simulink library "SDTlibV1"  (R2025b)
settings: Solver=VariableStepAuto  StartTime=0.0  StopTime=10.0  RelTol=1e-3
PreLoadFcn:
  | addpath(genpath('SDTfct'));
values from neighbouring files (symbols this model uses):
  pass = ra2DCMi(blk.ra)    [view_SDTlib_model.m]
undefined symbols (not defined in the file or in its folder): CMG, DAP0, DPa0, FSM, Ignew, InvDyn, InvDynAug, Jr, KIN, kinematic_model, LS, Mdyn, mnew, mp, OGnew, PMA, ra_norm, RWS, sig4, uls, ureal, uss, uw, XI
libraries: RCTblocks x470, $bdroot x4
(part 6 of 10)

== system SDTlibV1/Space  subsystems/Four CMGs Pyramid/P2//p' ==
  u : Inport  PortDimensions=18
  Demux : Demux  Outputs=[3 3 3 3 3 3]
  Mux : Mux  Inputs=[3 3 3 3 3 3]
  rotation : Gain  Gain=rot  Multiplication=Matrix(K*u) (u vector)
  rotation1 : Gain  Gain=rot  Multiplication=Matrix(K*u) (u vector)
  rotation2 : Gain  Gain=rot  Multiplication=Matrix(K*u) (u vector)
  translation : Gain  Gain=rot  Multiplication=Matrix(K*u) (u vector)
  translation1 : Gain  Gain=rot  Multiplication=Matrix(K*u) (u vector)
  translation2 : Gain  Gain=rot  Multiplication=Matrix(K*u) (u vector)
  y : Outport  VectorParamsAs1DForOutWhenUnconnected=off
  wires:
  rotation/1 -> Mux/2
  translation/1 -> Mux/1
  Demux/1 -> translation/1
  u/1 -> Demux/1
  Mux/1 -> y/1
  Demux/2 -> rotation/1
  Demux/4 -> rotation1/1
  Demux/3 -> translation1/1
  translation1/1 -> Mux/3
  rotation1/1 -> Mux/4
  Demux/5 -> translation2/1
  translation2/1 -> Mux/5
  rotation2/1 -> Mux/6
  Demux/6 -> rotation2/1

== system SDTlibV1/Space  subsystems/Four CMGs Pyramid/P3//p' ==
  u : Inport  PortDimensions=18
  Demux : Demux  Outputs=[3 3 3 3 3 3]
  Mux : Mux  Inputs=[3 3 3 3 3 3]
  rotation : Gain  Gain=rot  Multiplication=Matrix(K*u) (u vector)
  rotation1 : Gain  Gain=rot  Multiplication=Matrix(K*u) (u vector)
  rotation2 : Gain  Gain=rot  Multiplication=Matrix(K*u) (u vector)
  translation : Gain  Gain=rot  Multiplication=Matrix(K*u) (u vector)
  translation1 : Gain  Gain=rot  Multiplication=Matrix(K*u) (u vector)
  translation2 : Gain  Gain=rot  Multiplication=Matrix(K*u) (u vector)
  y : Outport  VectorParamsAs1DForOutWhenUnconnected=off
  wires:
  Demux/6 -> rotation2/1
  rotation2/1 -> Mux/6
  translation2/1 -> Mux/5
  Demux/5 -> translation2/1
  rotation1/1 -> Mux/4
  translation1/1 -> Mux/3
  Demux/3 -> translation1/1
  Demux/4 -> rotation1/1
  Demux/2 -> rotation/1
  Mux/1 -> y/1
  u/1 -> Demux/1
  Demux/1 -> translation/1
  translation/1 -> Mux/1
  rotation/1 -> Mux/2

== system SDTlibV1/Space  subsystems/Four CMGs Pyramid/P4//p' ==
  u : Inport  PortDimensions=18
  Demux : Demux  Outputs=[3 3 3 3 3 3]
  Mux : Mux  Inputs=[3 3 3 3 3 3]
  rotation : Gain  Gain=rot  Multiplication=Matrix(K*u) (u vector)
  rotation1 : Gain  Gain=rot  Multiplication=Matrix(K*u) (u vector)
  rotation2 : Gain  Gain=rot  Multiplication=Matrix(K*u) (u vector)
  translation : Gain  Gain=rot  Multiplication=Matrix(K*u) (u vector)
  translation1 : Gain  Gain=rot  Multiplication=Matrix(K*u) (u vector)
  translation2 : Gain  Gain=rot  Multiplication=Matrix(K*u) (u vector)
  y : Outport  VectorParamsAs1DForOutWhenUnconnected=off
  wires:
  rotation/1 -> Mux/2
  translation/1 -> Mux/1
  Demux/1 -> translation/1
  u/1 -> Demux/1
  Mux/1 -> y/1
  Demux/2 -> rotation/1
  Demux/4 -> rotation1/1
  Demux/3 -> translation1/1
  translation1/1 -> Mux/3
  rotation1/1 -> Mux/4
  Demux/5 -> translation2/1
  translation2/1 -> Mux/5
  rotation2/1 -> Mux/6
  Demux/6 -> rotation2/1

== system SDTlibV1/Space  subsystems/Four CMGs Pyramid/massless connection body ==
  in1 : Inport  PortDimensions=6
  in2 : Inport  Port=2  PortDimensions=6
  in3 : Inport  Port=3  PortDimensions=6
  in4 : Inport  Port=4  PortDimensions=6
  in5 : Inport  Port=5  PortDimensions=18
  Demux : Demux  Outputs=[ 18 18 18 18 6]
  Gain : RCTblocks/Uncertain State Space  Tag=USS  USystem=uss(KIN)  UValue=[]  X0=[]  uX0=[]
  Mux : Mux  Inputs=[ 6 6 6 6 18]
  out1 : Outport
  out2 : Outport  Port=2
  out3 : Outport  Port=3
  out4 : Outport  Port=4
  out5 : Outport  Port=5
  wires:
  Mux/1 -> Gain/1
  Gain/1 -> Demux/1
  in1/1 -> Mux/1
  Demux/1 -> out1/1
  in2/1 -> Mux/2
  Demux/2 -> out2/1
  in3/1 -> Mux/3
  Demux/3 -> out3/1
  in4/1 -> Mux/4
  Demux/4 -> out4/1
  in5/1 -> Mux/5
  Demux/5 -> out5/1

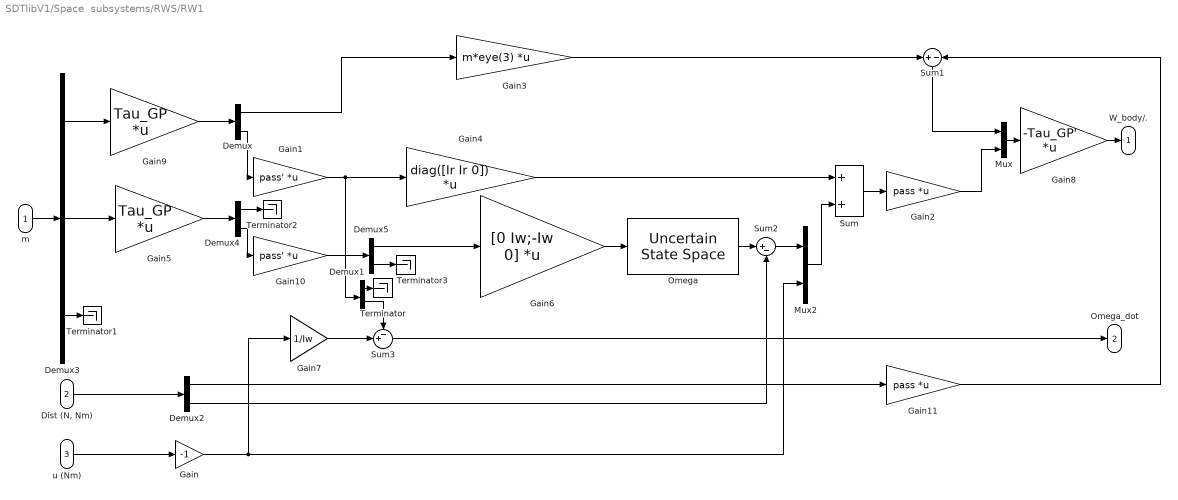
== system SDTlibV1/Space  subsystems/RWS/RW1 ==
  m : Inport  PortDimensions=18
  "Dist (N, Nm)    " : Inport  Port=2
  u (Nm) : Inport  Port=3  PortDimensions=1
  Demux : Demux  Outputs=[3 3]
  Demux1 : Demux  Outputs=[2 1]
  Demux2 : Demux  Outputs=[3 2]
  Demux3 : Demux  Outputs=[6 6 6]
  Demux4 : Demux  Outputs=[3 3]
  Demux5 : Demux  Outputs=[2 1]
  Gain : Gain  Gain=-1
  Gain1 : Gain  Gain=pass'  Multiplication=Matrix(K*u) (u vector)
  Gain10 : Gain  Gain=pass'  Multiplication=Matrix(K*u) (u vector)
  Gain11 : Gain  Gain=pass  Multiplication=Matrix(K*u) (u vector)
  Gain2 : Gain  Gain=pass  Multiplication=Matrix(K*u) (u vector)
  Gain3 : Gain  Gain=m*eye(3)  Multiplication=Matrix(K*u) (u vector)
  Gain4 : Gain  Gain=diag([Ir Ir 0])  Multiplication=Matrix(K*u) (u vector)
  Gain5 : Gain  Gain=Tau_GP  Multiplication=Matrix(K*u) (u vector)
  Gain6 : Gain  Gain=[0 Iw;-Iw 0]  Multiplication=Matrix(K*u) (u vector)
  Gain7 : Gain  Gain=1/Iw
  Gain8 : Gain  Gain=-Tau_GP'  Multiplication=Matrix(K*u) (u vector)
  Gain9 : Gain  Gain=Tau_GP  Multiplication=Matrix(K*u) (u vector)
  Mux : Mux  Inputs=[3 3]
  Mux2 : Mux  Inputs=[2 1]
  Omega : RCTblocks/Uncertain State Space  Tag=USS  USystem=uss(Omega*eye(2))  UValue=[]  X0=[]  uX0=[]
  Sum : Sum
  Sum1 : Sum  Inputs=+-
  Sum2 : Sum  Inputs=|+-
  Sum3 : Sum  Inputs=-+|
  Terminator{,1..3} (4 alike) : Terminator
  W_body/. : Outport  VectorParamsAs1DForOutWhenUnconnected=off
  Omega_dot : Outport  Port=2  PortDimensions=1  VectorParamsAs1DForOutWhenUnconnected=off
  wires:
  Sum3/1 -> Omega_dot/1
  Gain7/1 -> Sum3/2
  Mux2/1 -> Sum/2
  Sum2/1 -> Mux2/1
  Omega/1 -> Sum2/1
  Gain/1 -> Gain7/1, Mux2/2
  u (Nm)/1 -> Gain/1
  Sum1/1 -> Mux/1
  Gain11/1 -> Sum1/2
  Gain3/1 -> Sum1/1
  Demux2/2 -> Sum2/2
  "Dist (N, Nm)    "/1 -> Demux2/1
  Demux2/1 -> Gain11/1
  Gain9/1 -> Demux/1
  Mux/1 -> Gain8/1
  Gain8/1 -> W_body/./1
  Gain6/1 -> Omega/1
  Demux5/1 -> Gain6/1
  Gain1/1 -> Gain4/1, Demux1/1
  Sum/1 -> Gain2/1
  Gain4/1 -> Sum/1
  Demux/2 -> Gain1/1
  Demux/1 -> Gain3/1
  Gain2/1 -> Mux/2
  Demux3/1 -> Gain9/1
  m/1 -> Demux3/1
  Demux3/2 -> Gain5/1
  Demux1/2 -> Sum3/1
  Demux1/1 -> Terminator/1
  Demux3/3 -> Terminator1/1
  Demux4/2 -> Gain10/1
  Gain5/1 -> Demux4/1
  Demux4/1 -> Terminator2/1
  Gain10/1 -> Demux5/1
  Demux5/2 -> Terminator3/1

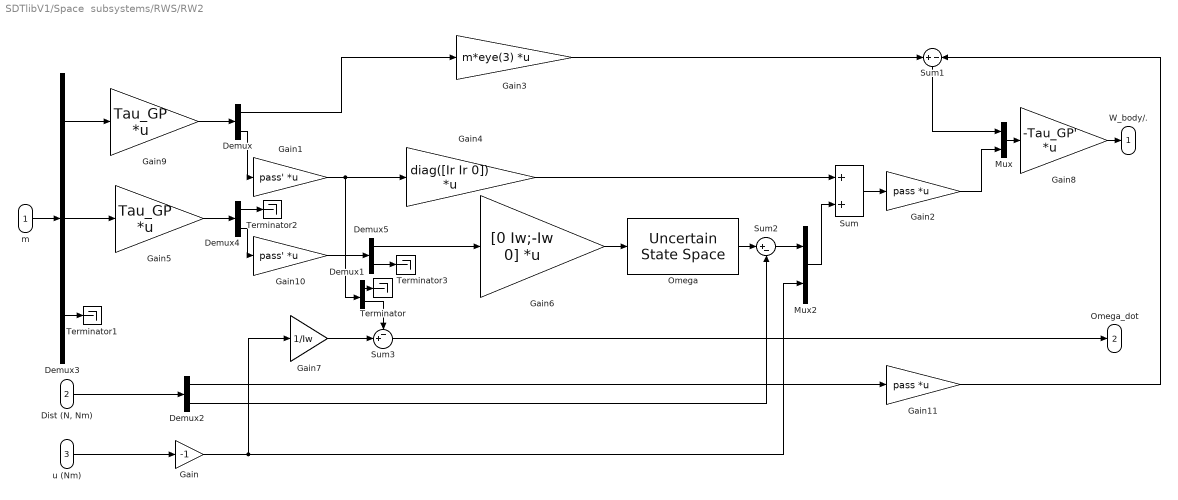
== system SDTlibV1/Space  subsystems/RWS/RW2 ==
  m : Inport  PortDimensions=18
  "Dist (N, Nm)    " : Inport  Port=2
  u (Nm) : Inport  Port=3  PortDimensions=1
  Demux : Demux  Outputs=[3 3]
  Demux1 : Demux  Outputs=[2 1]
  Demux2 : Demux  Outputs=[3 2]
  Demux3 : Demux  Outputs=[6 6 6]
  Demux4 : Demux  Outputs=[3 3]
  Demux5 : Demux  Outputs=[2 1]
  Gain : Gain  Gain=-1
  Gain1 : Gain  Gain=pass'  Multiplication=Matrix(K*u) (u vector)
  Gain10 : Gain  Gain=pass'  Multiplication=Matrix(K*u) (u vector)
  Gain11 : Gain  Gain=pass  Multiplication=Matrix(K*u) (u vector)
  Gain2 : Gain  Gain=pass  Multiplication=Matrix(K*u) (u vector)
  Gain3 : Gain  Gain=m*eye(3)  Multiplication=Matrix(K*u) (u vector)
  Gain4 : Gain  Gain=diag([Ir Ir 0])  Multiplication=Matrix(K*u) (u vector)
  Gain5 : Gain  Gain=Tau_GP  Multiplication=Matrix(K*u) (u vector)
  Gain6 : Gain  Gain=[0 Iw;-Iw 0]  Multiplication=Matrix(K*u) (u vector)
  Gain7 : Gain  Gain=1/Iw
  Gain8 : Gain  Gain=-Tau_GP'  Multiplication=Matrix(K*u) (u vector)
  Gain9 : Gain  Gain=Tau_GP  Multiplication=Matrix(K*u) (u vector)
  Mux : Mux  Inputs=[3 3]
  Mux2 : Mux  Inputs=[2 1]
  Omega : RCTblocks/Uncertain State Space  Tag=USS  USystem=uss(Omega*eye(2))  UValue=[]  X0=[]  uX0=[]
  Sum : Sum
  Sum1 : Sum  Inputs=+-
  Sum2 : Sum  Inputs=|+-
  Sum3 : Sum  Inputs=-+|
  Terminator{,1..3} (4 alike) : Terminator
  W_body/. : Outport  VectorParamsAs1DForOutWhenUnconnected=off
  Omega_dot : Outport  Port=2  PortDimensions=1  VectorParamsAs1DForOutWhenUnconnected=off
  wires:
  Demux5/2 -> Terminator3/1
  Gain10/1 -> Demux5/1
  Demux4/1 -> Terminator2/1
  Gain5/1 -> Demux4/1
  Demux4/2 -> Gain10/1
  Demux3/3 -> Terminator1/1
  Demux1/1 -> Terminator/1
  Demux1/2 -> Sum3/1
  Demux3/2 -> Gain5/1
  m/1 -> Demux3/1
  Demux3/1 -> Gain9/1
  Gain2/1 -> Mux/2
  Demux/1 -> Gain3/1
  Demux/2 -> Gain1/1
  Gain4/1 -> Sum/1
  Sum/1 -> Gain2/1
  Gain1/1 -> Demux1/1, Gain4/1
  Demux5/1 -> Gain6/1
  Gain6/1 -> Omega/1
  Gain8/1 -> W_body/./1
  Mux/1 -> Gain8/1
  Gain9/1 -> Demux/1
  Demux2/1 -> Gain11/1
  "Dist (N, Nm)    "/1 -> Demux2/1
  Demux2/2 -> Sum2/2
  Gain3/1 -> Sum1/1
  Gain11/1 -> Sum1/2
  Sum1/1 -> Mux/1
  u (Nm)/1 -> Gain/1
  Gain/1 -> Mux2/2, Gain7/1
  Omega/1 -> Sum2/1
  Sum2/1 -> Mux2/1
  Mux2/1 -> Sum/2
  Gain7/1 -> Sum3/2
  Sum3/1 -> Omega_dot/1

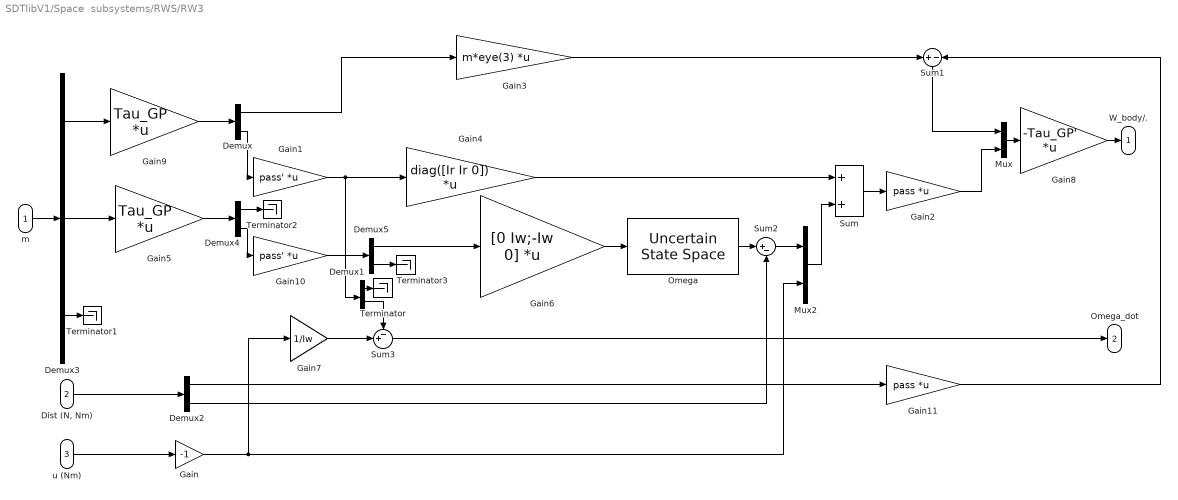
== system SDTlibV1/Space  subsystems/RWS/RW3 ==
  m : Inport  PortDimensions=18
  "Dist (N, Nm)    " : Inport  Port=2
  u (Nm) : Inport  Port=3  PortDimensions=1
  Demux : Demux  Outputs=[3 3]
  Demux1 : Demux  Outputs=[2 1]
  Demux2 : Demux  Outputs=[3 2]
  Demux3 : Demux  Outputs=[6 6 6]
  Demux4 : Demux  Outputs=[3 3]
  Demux5 : Demux  Outputs=[2 1]
  Gain : Gain  Gain=-1
  Gain1 : Gain  Gain=pass'  Multiplication=Matrix(K*u) (u vector)
  Gain10 : Gain  Gain=pass'  Multiplication=Matrix(K*u) (u vector)
  Gain11 : Gain  Gain=pass  Multiplication=Matrix(K*u) (u vector)
  Gain2 : Gain  Gain=pass  Multiplication=Matrix(K*u) (u vector)
  Gain3 : Gain  Gain=m*eye(3)  Multiplication=Matrix(K*u) (u vector)
  Gain4 : Gain  Gain=diag([Ir Ir 0])  Multiplication=Matrix(K*u) (u vector)
  Gain5 : Gain  Gain=Tau_GP  Multiplication=Matrix(K*u) (u vector)
  Gain6 : Gain  Gain=[0 Iw;-Iw 0]  Multiplication=Matrix(K*u) (u vector)
  Gain7 : Gain  Gain=1/Iw
  Gain8 : Gain  Gain=-Tau_GP'  Multiplication=Matrix(K*u) (u vector)
  Gain9 : Gain  Gain=Tau_GP  Multiplication=Matrix(K*u) (u vector)
  Mux : Mux  Inputs=[3 3]
  Mux2 : Mux  Inputs=[2 1]
  Omega : RCTblocks/Uncertain State Space  Tag=USS  USystem=uss(Omega*eye(2))  UValue=[]  X0=[]  uX0=[]
  Sum : Sum
  Sum1 : Sum  Inputs=+-
  Sum2 : Sum  Inputs=|+-
  Sum3 : Sum  Inputs=-+|
  Terminator{,1..3} (4 alike) : Terminator
  W_body/. : Outport  VectorParamsAs1DForOutWhenUnconnected=off
  Omega_dot : Outport  Port=2  PortDimensions=1  VectorParamsAs1DForOutWhenUnconnected=off
  wires:
  Sum3/1 -> Omega_dot/1
  Gain7/1 -> Sum3/2
  Mux2/1 -> Sum/2
  Sum2/1 -> Mux2/1
  Omega/1 -> Sum2/1
  Gain/1 -> Gain7/1, Mux2/2
  u (Nm)/1 -> Gain/1
  Sum1/1 -> Mux/1
  Gain11/1 -> Sum1/2
  Gain3/1 -> Sum1/1
  Demux2/2 -> Sum2/2
  "Dist (N, Nm)    "/1 -> Demux2/1
  Demux2/1 -> Gain11/1
  Gain9/1 -> Demux/1
  Mux/1 -> Gain8/1
  Gain8/1 -> W_body/./1
  Gain6/1 -> Omega/1
  Demux5/1 -> Gain6/1
  Gain1/1 -> Gain4/1, Demux1/1
  Sum/1 -> Gain2/1
  Gain4/1 -> Sum/1
  Demux/2 -> Gain1/1
  Demux/1 -> Gain3/1
  Gain2/1 -> Mux/2
  Demux3/1 -> Gain9/1
  m/1 -> Demux3/1
  Demux3/2 -> Gain5/1
  Demux1/2 -> Sum3/1
  Demux1/1 -> Terminator/1
  Demux3/3 -> Terminator1/1
  Demux4/2 -> Gain10/1
  Gain5/1 -> Demux4/1
  Demux4/1 -> Terminator2/1
  Gain10/1 -> Demux5/1
  Demux5/2 -> Terminator3/1

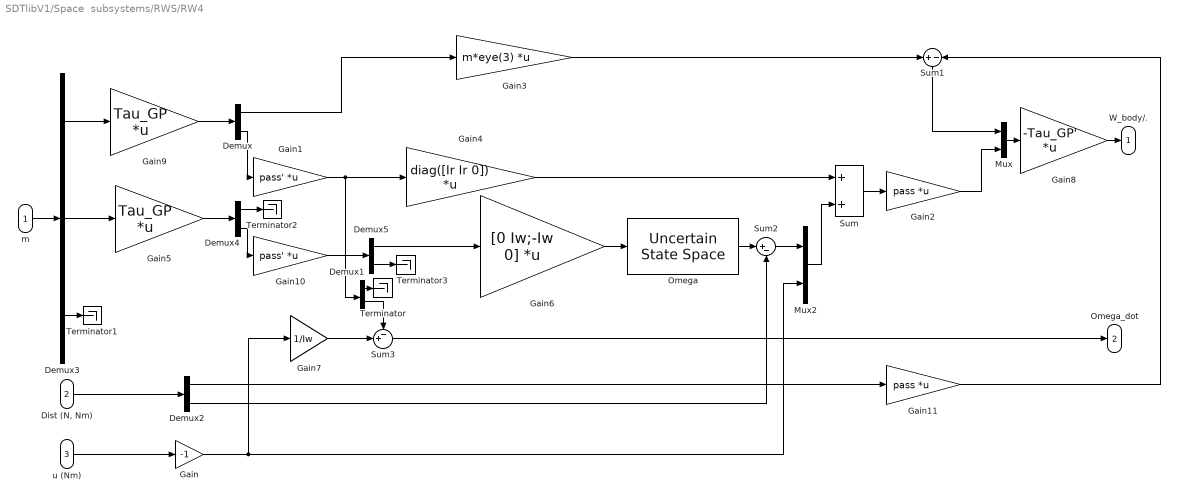
== system SDTlibV1/Space  subsystems/RWS/RW4 ==
  m : Inport  PortDimensions=18
  "Dist (N, Nm)    " : Inport  Port=2
  u (Nm) : Inport  Port=3  PortDimensions=1
  Demux : Demux  Outputs=[3 3]
  Demux1 : Demux  Outputs=[2 1]
  Demux2 : Demux  Outputs=[3 2]
  Demux3 : Demux  Outputs=[6 6 6]
  Demux4 : Demux  Outputs=[3 3]
  Demux5 : Demux  Outputs=[2 1]
  Gain : Gain  Gain=-1
  Gain1 : Gain  Gain=pass'  Multiplication=Matrix(K*u) (u vector)
  Gain10 : Gain  Gain=pass'  Multiplication=Matrix(K*u) (u vector)
  Gain11 : Gain  Gain=pass  Multiplication=Matrix(K*u) (u vector)
  Gain2 : Gain  Gain=pass  Multiplication=Matrix(K*u) (u vector)
  Gain3 : Gain  Gain=m*eye(3)  Multiplication=Matrix(K*u) (u vector)
  Gain4 : Gain  Gain=diag([Ir Ir 0])  Multiplication=Matrix(K*u) (u vector)
  Gain5 : Gain  Gain=Tau_GP  Multiplication=Matrix(K*u) (u vector)
  Gain6 : Gain  Gain=[0 Iw;-Iw 0]  Multiplication=Matrix(K*u) (u vector)
  Gain7 : Gain  Gain=1/Iw
  Gain8 : Gain  Gain=-Tau_GP'  Multiplication=Matrix(K*u) (u vector)
  Gain9 : Gain  Gain=Tau_GP  Multiplication=Matrix(K*u) (u vector)
  Mux : Mux  Inputs=[3 3]
  Mux2 : Mux  Inputs=[2 1]
  Omega : RCTblocks/Uncertain State Space  Tag=USS  USystem=uss(Omega*eye(2))  UValue=[]  X0=[]  uX0=[]
  Sum : Sum
  Sum1 : Sum  Inputs=+-
  Sum2 : Sum  Inputs=|+-
  Sum3 : Sum  Inputs=-+|
  Terminator{,1..3} (4 alike) : Terminator
  W_body/. : Outport  VectorParamsAs1DForOutWhenUnconnected=off
  Omega_dot : Outport  Port=2  PortDimensions=1  VectorParamsAs1DForOutWhenUnconnected=off
  wires:
  Demux5/2 -> Terminator3/1
  Gain10/1 -> Demux5/1
  Demux4/1 -> Terminator2/1
  Gain5/1 -> Demux4/1
  Demux4/2 -> Gain10/1
  Demux3/3 -> Terminator1/1
  Demux1/1 -> Terminator/1
  Demux1/2 -> Sum3/1
  Demux3/2 -> Gain5/1
  m/1 -> Demux3/1
  Demux3/1 -> Gain9/1
  Gain2/1 -> Mux/2
  Demux/1 -> Gain3/1
  Demux/2 -> Gain1/1
  Gain4/1 -> Sum/1
  Sum/1 -> Gain2/1
  Gain1/1 -> Demux1/1, Gain4/1
  Demux5/1 -> Gain6/1
  Gain6/1 -> Omega/1
  Gain8/1 -> W_body/./1
  Mux/1 -> Gain8/1
  Gain9/1 -> Demux/1
  Demux2/1 -> Gain11/1
  "Dist (N, Nm)    "/1 -> Demux2/1
  Demux2/2 -> Sum2/2
  Gain3/1 -> Sum1/1
  Gain11/1 -> Sum1/2
  Sum1/1 -> Mux/1
  u (Nm)/1 -> Gain/1
  Gain/1 -> Mux2/2, Gain7/1
  Omega/1 -> Sum2/1
  Sum2/1 -> Mux2/1
  Mux2/1 -> Sum/2
  Gain7/1 -> Sum3/2
  Sum3/1 -> Omega_dot/1

== system SDTlibV1/Space  subsystems/RWS/massless connection body ==
  in1 : Inport  PortDimensions=18
  in2 : Inport  Port=2  PortDimensions=6
  in3 : Inport  Port=3  PortDimensions=6
  in4 : Inport  Port=4  PortDimensions=6
  in5 : Inport  Port=5  PortDimensions=6
  Demux : Demux  Outputs=[ 6 18 18 18 18]
  Gain : RCTblocks/Uncertain State Space  Tag=USS  USystem=uss(KIN)  UValue=[]  X0=[]  uX0=[]
  Mux : Mux  Inputs=[ 18 6 6 6 6]
  out1 : Outport
  out2 : Outport  Port=2
  out3 : Outport  Port=3
  out4 : Outport  Port=4
  out5 : Outport  Port=5
  wires:
  Mux/1 -> Gain/1
  Gain/1 -> Demux/1
  in1/1 -> Mux/1
  Demux/1 -> out1/1
  in2/1 -> Mux/2
  Demux/2 -> out2/1
  in3/1 -> Mux/3
  Demux/3 -> out3/1
  in4/1 -> Mux/4
  Demux/4 -> out4/1
  in5/1 -> Mux/5
  Demux/5 -> out5/1

== system SDTlibV1/Space  subsystems/Set of 6 PMAss/18x18 DCM ==
  u : Inport  PortDimensions=18
  Demux : Demux  Outputs=[3 3 3 3 3 3]
  Mux : Mux  Inputs=[3 3 3 3 3 3]
  rotation : Gain  Gain=rot  Multiplication=Matrix(K*u) (u vector)
  rotation1 : Gain  Gain=rot  Multiplication=Matrix(K*u) (u vector)
  rotation2 : Gain  Gain=rot  Multiplication=Matrix(K*u) (u vector)
  translation : Gain  Gain=rot  Multiplication=Matrix(K*u) (u vector)
  translation1 : Gain  Gain=rot  Multiplication=Matrix(K*u) (u vector)
  translation2 : Gain  Gain=rot  Multiplication=Matrix(K*u) (u vector)
  y : Outport  VectorParamsAs1DForOutWhenUnconnected=off
  wires:
  rotation/1 -> Mux/2
  translation/1 -> Mux/1
  Demux/1 -> translation/1
  u/1 -> Demux/1
  Mux/1 -> y/1
  Demux/2 -> rotation/1
  Demux/4 -> rotation1/1
  Demux/3 -> translation1/1
  translation1/1 -> Mux/3
  rotation1/1 -> Mux/4
  Demux/5 -> translation2/1
  translation2/1 -> Mux/5
  rotation2/1 -> Mux/6
  Demux/6 -> rotation2/1

== system SDTlibV1/Space  subsystems/Set of 6 PMAss/18x18 DCM1 ==
  u : Inport  PortDimensions=18
  Demux : Demux  Outputs=[3 3 3 3 3 3]
  Mux : Mux  Inputs=[3 3 3 3 3 3]
  rotation : Gain  Gain=rot  Multiplication=Matrix(K*u) (u vector)
  rotation1 : Gain  Gain=rot  Multiplication=Matrix(K*u) (u vector)
  rotation2 : Gain  Gain=rot  Multiplication=Matrix(K*u) (u vector)
  translation : Gain  Gain=rot  Multiplication=Matrix(K*u) (u vector)
  translation1 : Gain  Gain=rot  Multiplication=Matrix(K*u) (u vector)
  translation2 : Gain  Gain=rot  Multiplication=Matrix(K*u) (u vector)
  y : Outport  VectorParamsAs1DForOutWhenUnconnected=off
  wires:
  Demux/6 -> rotation2/1
  rotation2/1 -> Mux/6
  translation2/1 -> Mux/5
  Demux/5 -> translation2/1
  rotation1/1 -> Mux/4
  translation1/1 -> Mux/3
  Demux/3 -> translation1/1
  Demux/4 -> rotation1/1
  Demux/2 -> rotation/1
  Mux/1 -> y/1
  u/1 -> Demux/1
  Demux/1 -> translation/1
  translation/1 -> Mux/1
  rotation/1 -> Mux/2

== system SDTlibV1/Space  subsystems/Set of 6 PMAss/18x18 DCM2 ==
  u : Inport  PortDimensions=18
  Demux : Demux  Outputs=[3 3 3 3 3 3]
  Mux : Mux  Inputs=[3 3 3 3 3 3]
  rotation : Gain  Gain=rot  Multiplication=Matrix(K*u) (u vector)
  rotation1 : Gain  Gain=rot  Multiplication=Matrix(K*u) (u vector)
  rotation2 : Gain  Gain=rot  Multiplication=Matrix(K*u) (u vector)
  translation : Gain  Gain=rot  Multiplication=Matrix(K*u) (u vector)
  translation1 : Gain  Gain=rot  Multiplication=Matrix(K*u) (u vector)
  translation2 : Gain  Gain=rot  Multiplication=Matrix(K*u) (u vector)
  y : Outport  VectorParamsAs1DForOutWhenUnconnected=off
  wires:
  rotation/1 -> Mux/2
  translation/1 -> Mux/1
  Demux/1 -> translation/1
  u/1 -> Demux/1
  Mux/1 -> y/1
  Demux/2 -> rotation/1
  Demux/4 -> rotation1/1
  Demux/3 -> translation1/1
  translation1/1 -> Mux/3
  rotation1/1 -> Mux/4
  Demux/5 -> translation2/1
  translation2/1 -> Mux/5
  rotation2/1 -> Mux/6
  Demux/6 -> rotation2/1

== system SDTlibV1/Space  subsystems/Set of 6 PMAss/6x6 DCM1 ==
  u : Inport  PortDimensions=6
  Demux : Demux  Outputs=[3 3]
  Mux : Mux  Inputs=[3 3]
  rotation : Gain  Gain=rot  Multiplication=Matrix(K*u) (u vector)
  translation : Gain  Gain=rot  Multiplication=Matrix(K*u) (u vector)
  y : Outport  VectorParamsAs1DForOutWhenUnconnected=off
  wires:
  rotation/1 -> Mux/2
  translation/1 -> Mux/1
  Demux/1 -> translation/1
  u/1 -> Demux/1
  Mux/1 -> y/1
  Demux/2 -> rotation/1

== system SDTlibV1/Space  subsystems/Set of 6 PMAss/6x6 DCM2 ==
  u : Inport  PortDimensions=6
  Demux : Demux  Outputs=[3 3]
  Mux : Mux  Inputs=[3 3]
  rotation : Gain  Gain=rot  Multiplication=Matrix(K*u) (u vector)
  translation : Gain  Gain=rot  Multiplication=Matrix(K*u) (u vector)
  y : Outport  VectorParamsAs1DForOutWhenUnconnected=off
  wires:
  rotation/1 -> Mux/2
  translation/1 -> Mux/1
  Demux/1 -> translation/1
  u/1 -> Demux/1
  Mux/1 -> y/1
  Demux/2 -> rotation/1

== system SDTlibV1/Space  subsystems/Set of 6 PMAss/6x6 DCM8 ==
  u : Inport  PortDimensions=6
  Demux : Demux  Outputs=[3 3]
  Mux : Mux  Inputs=[3 3]
  rotation : Gain  Gain=rot  Multiplication=Matrix(K*u) (u vector)
  translation : Gain  Gain=rot  Multiplication=Matrix(K*u) (u vector)
  y : Outport  VectorParamsAs1DForOutWhenUnconnected=off
  wires:
  Demux/2 -> rotation/1
  Mux/1 -> y/1
  u/1 -> Demux/1
  Demux/1 -> translation/1
  translation/1 -> Mux/1
  rotation/1 -> Mux/2

== system SDTlibV1/Space  subsystems/Set of 6 PMAss/PMA1 ==
  m_P : Inport
  u_PMA : Inport  Port=2
  Demux : Demux  Outputs=[6 12]
  Multi port rigid body : Subsystem  mask(Multi-port rigid body (6nx6n)){m=Mc-mp, Ig=IatG, OG=PG, n=2, numinv=1, OP1=[0;0;0], OP2=PG, OP3=[ureal('P3_y',1,'percent',10);0;0], OP4=[0;0;0], OP5=[0;0;0]}
      mask prompts: m "Mass (Kg)"; Ig "Inertia (at G, Kg m^2)"; OG "OG (3x1 vector, m)"; n "Number of ports"; numinv "Port to be inverted"; OP1 "OP1 (3x1 vector, m)"; OP2 "OP2 (3x1 vector, m)"; OP3 "OP3 (3x1 vector, m)"; OP4 "OP4 (3x1 vector, m)"; OP5 "OP5 (3x1 vector,m)"
      mask help:
      | 6nx6n dynamic model of a rigid body at n given points (ports) between wrenches applied at the n points (input) and acceleration twists at these points (output).
      |
      | 0: the reference point
      | G: the center of mass
      | Pi (i=1:n): the n given connection points (n<6).
      |
      | All parameters are expressed in the body frame.
      | Each parameter can be an uncertain parameter declared with "ureal"
      |
      | The 6x6 channel associated to one port can be inverted: then the input of this channel is the acceleration twist imposed at this point and the output is the wrench applied by this body.
      mask init:
      | MultiPortRigidBodyAug
      mask Help: web('Docmultiportrigidbody.html','-browser','-browser')
      mask TypeOptions n: 1 | 2 | 3 | 4 | 5
      mask TypeOptions numinv: 1 | 2 | 3 | 4 | 5
      mask DialogControl ParameterGroupVar Prompt: Main parameters
      mask DialogControl port1 Prompt: Port #1
      mask DialogControl port2 Prompt: #2
      mask DialogControl port3 Prompt: #3
      mask DialogControl port4 Prompt: #4
      mask DialogControl port5 Prompt: #5
      mask Display:
      | disp('Multi-port\n rigid body\n [18(n-1)+6]x[6(n-1)+18])')
      | if n==1,
      |     if numinv==1,
      |         port_label('input', 1,'m_P')
      |         port_label('output',1,'W_body/.,P')
      |     else
      |         port_label('input', 1,'W_./body,P')
      |         port_label('output',1,'m_P')
      |     end
      | else
      |     for ii=1:n
      |         if numinv==ii,
      |             port_label('output',ii,['W_body/.,P',num2str(ii)])
      |             port_label('input', ii,['m_P',num2str(ii)])
      |         else
      |             port_label('input', ii,['W_./body,P',num2str(ii)])
      |             port_label('output',ii,['m_P',num2str(ii)])
      |         end
      |     end
      | end
  Terminator : Terminator
  proof mass : Subsystem  mask(Mass-spring-model model(6x6)){v=v, m=mp, k=k, d=d}
      mask prompts: v "v (3x1 vector)"; m "mass (Kg)"; k "stiffness (N/m)"; d "damper (Ns/m)"
      mask help:
      | Simplified dynamic model of a spring-mass-damper model located at point P (connection point with the hub):
      | 6x6 transfer between acceleretion twist at P and wrench applied by the spring-mass system at P. The model is expressed in the (inherit) body frame.
      |
      | v: the direction vector of the spring-mass system.
      | Each parameter (except v) can be an uncertain parameter declared with "ureal"
      mask init:
      | pass=ra2DCMi(v);
      mask DialogControl ParameterGroupVar Prompt: Main parameters
      mask Display:
      | disp('1D \n mass-spring-damper \n model(6x6)')
      | port_label('input', 1, 'Xddot')
      | port_label('output', 1, 'W_body/.')
      | port_label('input', 2, 'u_PMA')
      | port_label('output', 2, 'x_PMA')
  W_body/.,P : Outport
  x_PMA : Outport  Port=2
  wires:
  Multi port rigid body/1(out1) -> W_body/.,P/1
  u_PMA/1 -> proof mass/2(u_PMA)
  m_P/1 -> Multi port rigid body/1(in1)
  proof mass/1(W_body/.) -> Multi port rigid body/2(in2)
  proof mass/2(x_PMA) -> x_PMA/1
  Multi port rigid body/2(out2) -> Demux/1
  Demux/1 -> proof mass/1(Xddot)
  Demux/2 -> Terminator/1

== system SDTlibV1/Space  subsystems/Set of 6 PMAss/PMA2 ==
  m_P : Inport
  u_PMA : Inport  Port=2
  Demux : Demux  Outputs=[6 12]
  Multi port rigid body : Subsystem  mask(Multi-port rigid body (6nx6n)){m=Mc-mp, Ig=IatG, OG=PG, n=2, numinv=1, OP1=[0;0;0], OP2=PG, OP3=[ureal('P3_y',1,'percent',10);0;0], OP4=[0;0;0], OP5=[0;0;0]}
      mask prompts: m "Mass (Kg)"; Ig "Inertia (at G, Kg m^2)"; OG "OG (3x1 vector, m)"; n "Number of ports"; numinv "Port to be inverted"; OP1 "OP1 (3x1 vector, m)"; OP2 "OP2 (3x1 vector, m)"; OP3 "OP3 (3x1 vector, m)"; OP4 "OP4 (3x1 vector, m)"; OP5 "OP5 (3x1 vector,m)"
      mask help:
      | 6nx6n dynamic model of a rigid body at n given points (ports) between wrenches applied at the n points (input) and acceleration twists at these points (output).
      |
      | 0: the reference point
      | G: the center of mass
      | Pi (i=1:n): the n given connection points (n<6).
      |
      | All parameters are expressed in the body frame.
      | Each parameter can be an uncertain parameter declared with "ureal"
      |
      | The 6x6 channel associated to one port can be inverted: then the input of this channel is the acceleration twist imposed at this point and the output is the wrench applied by this body.
      mask init:
      | MultiPortRigidBodyAug
      mask Help: web('Docmultiportrigidbody.html','-browser','-browser')
      mask TypeOptions n: 1 | 2 | 3 | 4 | 5
      mask TypeOptions numinv: 1 | 2 | 3 | 4 | 5
      mask DialogControl ParameterGroupVar Prompt: Main parameters
      mask DialogControl port1 Prompt: Port #1
      mask DialogControl port2 Prompt: #2
      mask DialogControl port3 Prompt: #3
      mask DialogControl port4 Prompt: #4
      mask DialogControl port5 Prompt: #5
      mask Display:
      | disp('Multi-port\n rigid body\n [18(n-1)+6]x[6(n-1)+18])')
      | if n==1,
      |     if numinv==1,
      |         port_label('input', 1,'m_P')
      |         port_label('output',1,'W_body/.,P')
      |     else
      |         port_label('input', 1,'W_./body,P')
      |         port_label('output',1,'m_P')
      |     end
      | else
      |     for ii=1:n
      |         if numinv==ii,
      |             port_label('output',ii,['W_body/.,P',num2str(ii)])
      |             port_label('input', ii,['m_P',num2str(ii)])
      |         else
      |             port_label('input', ii,['W_./body,P',num2str(ii)])
      |             port_label('output',ii,['m_P',num2str(ii)])
      |         end
      |     end
      | end
  Terminator : Terminator
  proof mass : Subsystem  mask(Mass-spring-model model(6x6)){v=v, m=mp, k=k, d=d}
      mask prompts: v "v (3x1 vector)"; m "mass (Kg)"; k "stiffness (N/m)"; d "damper (Ns/m)"
      mask help:
      | Simplified dynamic model of a spring-mass-damper model located at point P (connection point with the hub):
      | 6x6 transfer between acceleretion twist at P and wrench applied by the spring-mass system at P. The model is expressed in the (inherit) body frame.
      |
      | v: the direction vector of the spring-mass system.
      | Each parameter (except v) can be an uncertain parameter declared with "ureal"
      mask init:
      | pass=ra2DCMi(v);
      mask DialogControl ParameterGroupVar Prompt: Main parameters
      mask Display:
      | disp('1D \n mass-spring-damper \n model(6x6)')
      | port_label('input', 1, 'Xddot')
      | port_label('output', 1, 'W_body/.')
      | port_label('input', 2, 'u_PMA')
      | port_label('output', 2, 'x_PMA')
  W_body/.,P : Outport
  x_PMA : Outport  Port=2
  wires:
  Demux/2 -> Terminator/1
  Demux/1 -> proof mass/1(Xddot)
  Multi port rigid body/2(out2) -> Demux/1
  proof mass/2(x_PMA) -> x_PMA/1
  proof mass/1(W_body/.) -> Multi port rigid body/2(in2)
  m_P/1 -> Multi port rigid body/1(in1)
  u_PMA/1 -> proof mass/2(u_PMA)
  Multi port rigid body/1(out1) -> W_body/.,P/1

== system SDTlibV1/Space  subsystems/Set of 6 PMAss/PMA3 ==
  m_P : Inport
  u_PMA : Inport  Port=2
  Demux : Demux  Outputs=[6 12]
  Multi port rigid body : Subsystem  mask(Multi-port rigid body (6nx6n)){m=Mc-mp, Ig=IatG, OG=PG, n=2, numinv=1, OP1=[0;0;0], OP2=PG, OP3=[ureal('P3_y',1,'percent',10);0;0], OP4=[0;0;0], OP5=[0;0;0]}
      mask prompts: m "Mass (Kg)"; Ig "Inertia (at G, Kg m^2)"; OG "OG (3x1 vector, m)"; n "Number of ports"; numinv "Port to be inverted"; OP1 "OP1 (3x1 vector, m)"; OP2 "OP2 (3x1 vector, m)"; OP3 "OP3 (3x1 vector, m)"; OP4 "OP4 (3x1 vector, m)"; OP5 "OP5 (3x1 vector,m)"
      mask help:
      | 6nx6n dynamic model of a rigid body at n given points (ports) between wrenches applied at the n points (input) and acceleration twists at these points (output).
      |
      | 0: the reference point
      | G: the center of mass
      | Pi (i=1:n): the n given connection points (n<6).
      |
      | All parameters are expressed in the body frame.
      | Each parameter can be an uncertain parameter declared with "ureal"
      |
      | The 6x6 channel associated to one port can be inverted: then the input of this channel is the acceleration twist imposed at this point and the output is the wrench applied by this body.
      mask init:
      | MultiPortRigidBodyAug
      mask Help: web('Docmultiportrigidbody.html','-browser','-browser')
      mask TypeOptions n: 1 | 2 | 3 | 4 | 5
      mask TypeOptions numinv: 1 | 2 | 3 | 4 | 5
      mask DialogControl ParameterGroupVar Prompt: Main parameters
      mask DialogControl port1 Prompt: Port #1
      mask DialogControl port2 Prompt: #2
      mask DialogControl port3 Prompt: #3
      mask DialogControl port4 Prompt: #4
      mask DialogControl port5 Prompt: #5
      mask Display:
      | disp('Multi-port\n rigid body\n [18(n-1)+6]x[6(n-1)+18])')
      | if n==1,
      |     if numinv==1,
      |         port_label('input', 1,'m_P')
      |         port_label('output',1,'W_body/.,P')
      |     else
      |         port_label('input', 1,'W_./body,P')
      |         port_label('output',1,'m_P')
      |     end
      | else
      |     for ii=1:n
      |         if numinv==ii,
      |             port_label('output',ii,['W_body/.,P',num2str(ii)])
      |             port_label('input', ii,['m_P',num2str(ii)])
      |         else
      |             port_label('input', ii,['W_./body,P',num2str(ii)])
      |             port_label('output',ii,['m_P',num2str(ii)])
      |         end
      |     end
      | end
  Terminator : Terminator
  proof mass : Subsystem  mask(Mass-spring-model model(6x6)){v=v, m=mp, k=k, d=d}
      mask prompts: v "v (3x1 vector)"; m "mass (Kg)"; k "stiffness (N/m)"; d "damper (Ns/m)"
      mask help:
      | Simplified dynamic model of a spring-mass-damper model located at point P (connection point with the hub):
      | 6x6 transfer between acceleretion twist at P and wrench applied by the spring-mass system at P. The model is expressed in the (inherit) body frame.
      |
      | v: the direction vector of the spring-mass system.
      | Each parameter (except v) can be an uncertain parameter declared with "ureal"
      mask init:
      | pass=ra2DCMi(v);
      mask DialogControl ParameterGroupVar Prompt: Main parameters
      mask Display:
      | disp('1D \n mass-spring-damper \n model(6x6)')
      | port_label('input', 1, 'Xddot')
      | port_label('output', 1, 'W_body/.')
      | port_label('input', 2, 'u_PMA')
      | port_label('output', 2, 'x_PMA')
  W_body/.,P : Outport
  x_PMA : Outport  Port=2
  wires:
  Multi port rigid body/1(out1) -> W_body/.,P/1
  u_PMA/1 -> proof mass/2(u_PMA)
  m_P/1 -> Multi port rigid body/1(in1)
  proof mass/1(W_body/.) -> Multi port rigid body/2(in2)
  proof mass/2(x_PMA) -> x_PMA/1
  Multi port rigid body/2(out2) -> Demux/1
  Demux/1 -> proof mass/1(Xddot)
  Demux/2 -> Terminator/1

== system SDTlibV1/Space  subsystems/Set of 6 PMAss/PMA4 ==
  m_P : Inport
  u_PMA : Inport  Port=2
  Demux : Demux  Outputs=[6 12]
  Multi port rigid body : Subsystem  mask(Multi-port rigid body (6nx6n)){m=Mc-mp, Ig=IatG, OG=PG, n=2, numinv=1, OP1=[0;0;0], OP2=PG, OP3=[ureal('P3_y',1,'percent',10);0;0], OP4=[0;0;0], OP5=[0;0;0]}
      mask prompts: m "Mass (Kg)"; Ig "Inertia (at G, Kg m^2)"; OG "OG (3x1 vector, m)"; n "Number of ports"; numinv "Port to be inverted"; OP1 "OP1 (3x1 vector, m)"; OP2 "OP2 (3x1 vector, m)"; OP3 "OP3 (3x1 vector, m)"; OP4 "OP4 (3x1 vector, m)"; OP5 "OP5 (3x1 vector,m)"
      mask help:
      | 6nx6n dynamic model of a rigid body at n given points (ports) between wrenches applied at the n points (input) and acceleration twists at these points (output).
      |
      | 0: the reference point
      | G: the center of mass
      | Pi (i=1:n): the n given connection points (n<6).
      |
      | All parameters are expressed in the body frame.
      | Each parameter can be an uncertain parameter declared with "ureal"
      |
      | The 6x6 channel associated to one port can be inverted: then the input of this channel is the acceleration twist imposed at this point and the output is the wrench applied by this body.
      mask init:
      | MultiPortRigidBodyAug
      mask Help: web('Docmultiportrigidbody.html','-browser','-browser')
      mask TypeOptions n: 1 | 2 | 3 | 4 | 5
      mask TypeOptions numinv: 1 | 2 | 3 | 4 | 5
      mask DialogControl ParameterGroupVar Prompt: Main parameters
      mask DialogControl port1 Prompt: Port #1
      mask DialogControl port2 Prompt: #2
      mask DialogControl port3 Prompt: #3
      mask DialogControl port4 Prompt: #4
      mask DialogControl port5 Prompt: #5
      mask Display:
      | disp('Multi-port\n rigid body\n [18(n-1)+6]x[6(n-1)+18])')
      | if n==1,
      |     if numinv==1,
      |         port_label('input', 1,'m_P')
      |         port_label('output',1,'W_body/.,P')
      |     else
      |         port_label('input', 1,'W_./body,P')
      |         port_label('output',1,'m_P')
      |     end
      | else
      |     for ii=1:n
      |         if numinv==ii,
      |             port_label('output',ii,['W_body/.,P',num2str(ii)])
      |             port_label('input', ii,['m_P',num2str(ii)])
      |         else
      |             port_label('input', ii,['W_./body,P',num2str(ii)])
      |             port_label('output',ii,['m_P',num2str(ii)])
      |         end
      |     end
      | end
  Terminator : Terminator
  proof mass : Subsystem  mask(Mass-spring-model model(6x6)){v=v, m=mp, k=k, d=d}
      mask prompts: v "v (3x1 vector)"; m "mass (Kg)"; k "stiffness (N/m)"; d "damper (Ns/m)"
      mask help:
      | Simplified dynamic model of a spring-mass-damper model located at point P (connection point with the hub):
      | 6x6 transfer between acceleretion twist at P and wrench applied by the spring-mass system at P. The model is expressed in the (inherit) body frame.
      |
      | v: the direction vector of the spring-mass system.
      | Each parameter (except v) can be an uncertain parameter declared with "ureal"
      mask init:
      | pass=ra2DCMi(v);
      mask DialogControl ParameterGroupVar Prompt: Main parameters
      mask Display:
      | disp('1D \n mass-spring-damper \n model(6x6)')
      | port_label('input', 1, 'Xddot')
      | port_label('output', 1, 'W_body/.')
      | port_label('input', 2, 'u_PMA')
      | port_label('output', 2, 'x_PMA')
  W_body/.,P : Outport
  x_PMA : Outport  Port=2
  wires:
  Demux/2 -> Terminator/1
  Demux/1 -> proof mass/1(Xddot)
  Multi port rigid body/2(out2) -> Demux/1
  proof mass/2(x_PMA) -> x_PMA/1
  proof mass/1(W_body/.) -> Multi port rigid body/2(in2)
  m_P/1 -> Multi port rigid body/1(in1)
  u_PMA/1 -> proof mass/2(u_PMA)
  Multi port rigid body/1(out1) -> W_body/.,P/1

== system SDTlibV1/Space  subsystems/Set of 6 PMAss/PMA5 ==
  m_P : Inport
  u_PMA : Inport  Port=2
  Demux : Demux  Outputs=[6 12]
  Multi port rigid body : Subsystem  mask(Multi-port rigid body (6nx6n)){m=Mc-mp, Ig=IatG, OG=PG, n=2, numinv=1, OP1=[0;0;0], OP2=PG, OP3=[ureal('P3_y',1,'percent',10);0;0], OP4=[0;0;0], OP5=[0;0;0]}
      mask prompts: m "Mass (Kg)"; Ig "Inertia (at G, Kg m^2)"; OG "OG (3x1 vector, m)"; n "Number of ports"; numinv "Port to be inverted"; OP1 "OP1 (3x1 vector, m)"; OP2 "OP2 (3x1 vector, m)"; OP3 "OP3 (3x1 vector, m)"; OP4 "OP4 (3x1 vector, m)"; OP5 "OP5 (3x1 vector,m)"
      mask help:
      | 6nx6n dynamic model of a rigid body at n given points (ports) between wrenches applied at the n points (input) and acceleration twists at these points (output).
      |
      | 0: the reference point
      | G: the center of mass
      | Pi (i=1:n): the n given connection points (n<6).
      |
      | All parameters are expressed in the body frame.
      | Each parameter can be an uncertain parameter declared with "ureal"
      |
      | The 6x6 channel associated to one port can be inverted: then the input of this channel is the acceleration twist imposed at this point and the output is the wrench applied by this body.
      mask init:
      | MultiPortRigidBodyAug
      mask Help: web('Docmultiportrigidbody.html','-browser','-browser')
      mask TypeOptions n: 1 | 2 | 3 | 4 | 5
      mask TypeOptions numinv: 1 | 2 | 3 | 4 | 5
      mask DialogControl ParameterGroupVar Prompt: Main parameters
      mask DialogControl port1 Prompt: Port #1
      mask DialogControl port2 Prompt: #2
      mask DialogControl port3 Prompt: #3
      mask DialogControl port4 Prompt: #4
      mask DialogControl port5 Prompt: #5
      mask Display:
      | disp('Multi-port\n rigid body\n [18(n-1)+6]x[6(n-1)+18])')
      | if n==1,
      |     if numinv==1,
      |         port_label('input', 1,'m_P')
      |         port_label('output',1,'W_body/.,P')
      |     else
      |         port_label('input', 1,'W_./body,P')
      |         port_label('output',1,'m_P')
      |     end
      | else
      |     for ii=1:n
      |         if numinv==ii,
      |             port_label('output',ii,['W_body/.,P',num2str(ii)])
      |             port_label('input', ii,['m_P',num2str(ii)])
      |         else
      |             port_label('input', ii,['W_./body,P',num2str(ii)])
      |             port_label('output',ii,['m_P',num2str(ii)])
      |         end
      |     end
      | end
  Terminator : Terminator
  proof mass : Subsystem  mask(Mass-spring-model model(6x6)){v=v, m=mp, k=k, d=d}
      mask prompts: v "v (3x1 vector)"; m "mass (Kg)"; k "stiffness (N/m)"; d "damper (Ns/m)"
      mask help:
      | Simplified dynamic model of a spring-mass-damper model located at point P (connection point with the hub):
      | 6x6 transfer between acceleretion twist at P and wrench applied by the spring-mass system at P. The model is expressed in the (inherit) body frame.
      |
      | v: the direction vector of the spring-mass system.
      | Each parameter (except v) can be an uncertain parameter declared with "ureal"
      mask init:
      | pass=ra2DCMi(v);
      mask DialogControl ParameterGroupVar Prompt: Main parameters
      mask Display:
      | disp('1D \n mass-spring-damper \n model(6x6)')
      | port_label('input', 1, 'Xddot')
      | port_label('output', 1, 'W_body/.')
      | port_label('input', 2, 'u_PMA')
      | port_label('output', 2, 'x_PMA')
  W_body/.,P : Outport
  x_PMA : Outport  Port=2
  wires:
  Multi port rigid body/1(out1) -> W_body/.,P/1
  u_PMA/1 -> proof mass/2(u_PMA)
  m_P/1 -> Multi port rigid body/1(in1)
  proof mass/1(W_body/.) -> Multi port rigid body/2(in2)
  proof mass/2(x_PMA) -> x_PMA/1
  Multi port rigid body/2(out2) -> Demux/1
  Demux/1 -> proof mass/1(Xddot)
  Demux/2 -> Terminator/1

== system SDTlibV1/Space  subsystems/Set of 6 PMAss/PMA6 ==
  m_P : Inport
  u_PMA : Inport  Port=2
  Demux : Demux  Outputs=[6 12]
  Multi port rigid body : Subsystem  mask(Multi-port rigid body (6nx6n)){m=Mc-mp, Ig=IatG, OG=PG, n=2, numinv=1, OP1=[0;0;0], OP2=PG, OP3=[ureal('P3_y',1,'percent',10);0;0], OP4=[0;0;0], OP5=[0;0;0]}
      mask prompts: m "Mass (Kg)"; Ig "Inertia (at G, Kg m^2)"; OG "OG (3x1 vector, m)"; n "Number of ports"; numinv "Port to be inverted"; OP1 "OP1 (3x1 vector, m)"; OP2 "OP2 (3x1 vector, m)"; OP3 "OP3 (3x1 vector, m)"; OP4 "OP4 (3x1 vector, m)"; OP5 "OP5 (3x1 vector,m)"
      mask help:
      | 6nx6n dynamic model of a rigid body at n given points (ports) between wrenches applied at the n points (input) and acceleration twists at these points (output).
      |
      | 0: the reference point
      | G: the center of mass
      | Pi (i=1:n): the n given connection points (n<6).
      |
      | All parameters are expressed in the body frame.
      | Each parameter can be an uncertain parameter declared with "ureal"
      |
      | The 6x6 channel associated to one port can be inverted: then the input of this channel is the acceleration twist imposed at this point and the output is the wrench applied by this body.
      mask init:
      | MultiPortRigidBodyAug
      mask Help: web('Docmultiportrigidbody.html','-browser','-browser')
      mask TypeOptions n: 1 | 2 | 3 | 4 | 5
      mask TypeOptions numinv: 1 | 2 | 3 | 4 | 5
      mask DialogControl ParameterGroupVar Prompt: Main parameters
      mask DialogControl port1 Prompt: Port #1
      mask DialogControl port2 Prompt: #2
      mask DialogControl port3 Prompt: #3
      mask DialogControl port4 Prompt: #4
      mask DialogControl port5 Prompt: #5
      mask Display:
      | disp('Multi-port\n rigid body\n [18(n-1)+6]x[6(n-1)+18])')
      | if n==1,
      |     if numinv==1,
      |         port_label('input', 1,'m_P')
      |         port_label('output',1,'W_body/.,P')
      |     else
      |         port_label('input', 1,'W_./body,P')
      |         port_label('output',1,'m_P')
      |     end
      | else
      |     for ii=1:n
      |         if numinv==ii,
      |             port_label('output',ii,['W_body/.,P',num2str(ii)])
      |             port_label('input', ii,['m_P',num2str(ii)])
      |         else
      |             port_label('input', ii,['W_./body,P',num2str(ii)])
      |             port_label('output',ii,['m_P',num2str(ii)])
      |         end
      |     end
      | end
  Terminator : Terminator
  proof mass : Subsystem  mask(Mass-spring-model model(6x6)){v=v, m=mp, k=k, d=d}
      mask prompts: v "v (3x1 vector)"; m "mass (Kg)"; k "stiffness (N/m)"; d "damper (Ns/m)"
      mask help:
      | Simplified dynamic model of a spring-mass-damper model located at point P (connection point with the hub):
      | 6x6 transfer between acceleretion twist at P and wrench applied by the spring-mass system at P. The model is expressed in the (inherit) body frame.
      |
      | v: the direction vector of the spring-mass system.
      | Each parameter (except v) can be an uncertain parameter declared with "ureal"
      mask init:
      | pass=ra2DCMi(v);
      mask DialogControl ParameterGroupVar Prompt: Main parameters
      mask Display:
      | disp('1D \n mass-spring-damper \n model(6x6)')
      | port_label('input', 1, 'Xddot')
      | port_label('output', 1, 'W_body/.')
      | port_label('input', 2, 'u_PMA')
      | port_label('output', 2, 'x_PMA')
  W_body/.,P : Outport
  x_PMA : Outport  Port=2
  wires:
  Demux/2 -> Terminator/1
  Demux/1 -> proof mass/1(Xddot)
  Multi port rigid body/2(out2) -> Demux/1
  proof mass/2(x_PMA) -> x_PMA/1
  proof mass/1(W_body/.) -> Multi port rigid body/2(in2)
  m_P/1 -> Multi port rigid body/1(in1)
  u_PMA/1 -> proof mass/2(u_PMA)
  Multi port rigid body/1(out1) -> W_body/.,P/1

== system SDTlibV1/Space  subsystems/Set of 6 PMAss/massless connection body ==
  in1 : Inport  PortDimensions=18
  in2 : Inport  Port=2  PortDimensions=6
  in3 : Inport  Port=3  PortDimensions=6
  in4 : Inport  Port=4  PortDimensions=6
  in5 : Inport  Port=5  PortDimensions=6
  in6 : Inport  Port=6  PortDimensions=6
  in7 : Inport  Port=7  PortDimensions=6
  Demux : Demux  Outputs=[ 6 18 18 18 18 18 18]
  Gain : RCTblocks/Uncertain State Space  Tag=USS  USystem=uss(KIN)  UValue=[]  X0=[]  uX0=[]
  Mux : Mux  Inputs=[ 18 6 6 6 6 6 6]
  out1 : Outport
  out2 : Outport  Port=2
  out3 : Outport  Port=3
  out4 : Outport  Port=4
  out5 : Outport  Port=5
  out6 : Outport  Port=6
  out7 : Outport  Port=7
  wires:
  Mux/1 -> Gain/1
  Gain/1 -> Demux/1
  in1/1 -> Mux/1
  Demux/1 -> out1/1
  in2/1 -> Mux/2
  Demux/2 -> out2/1
  in3/1 -> Mux/3
  Demux/3 -> out3/1
  in4/1 -> Mux/4
  Demux/4 -> out4/1
  in5/1 -> Mux/5
  Demux/5 -> out5/1
  in6/1 -> Mux/6
  Demux/6 -> out6/1
  in7/1 -> Mux/7
  Demux/7 -> out7/1

== system SDTlibV1/6 dof mechanisms/Revolute joint + configuration/18x18 v-u_rotation/Subsystem ==
  In1 : Inport
  Demux : Demux  Outputs=3
  Gain : Gain  Gain=2
  Gain1 : Gain  Gain=-2
  Gain2 : Gain  Gain=2
  Gain3 : Gain  Gain=2
  Gain4 : Gain  Gain=pass  Multiplication=Matrix(K*u) (u vector)
  Gain5 : Gain  Gain=pass'  Multiplication=Matrix(K*u) (u vector)
  Mux : Mux  Inputs=3
  Sum : Sum  Inputs=++|
  Sum1 : Sum  Inputs=|++
  Sum2 : Sum  Inputs=|+-
  Sum3 : Sum  Inputs=|++
  Sum4 : Sum  Inputs=++|
  Sum5 : Sum  Inputs=++|
  Uncertain State Space{,1..3} (4 alike) : RCTblocks/Uncertain State Space  Tag=USS  USystem=uss(sig4)  UValue=[]  X0=[]  uX0=[]
  Out1 : Outport  VectorParamsAs1DForOutWhenUnconnected=off
  wires:
  Gain5/1 -> Demux/1
  Gain4/1 -> Out1/1
  Uncertain State Space3/1 -> Sum3/2
  Gain2/1 -> Sum3/1
  In1/1 -> Gain5/1
  Gain/1 -> Sum/2
  Uncertain State Space2/1 -> Uncertain State Space3/1, Sum4/2, Sum2/2
  Demux/1 -> Gain3/1, Sum1/2
  Demux/3 -> Mux/3
  Mux/1 -> Gain4/1
  Sum4/1 -> Mux/2
  Sum3/1 -> Uncertain State Space2/1
  Gain1/1 -> Sum2/1
  Uncertain State Space/1 -> Uncertain State Space1/1, Sum5/1, Sum1/1
  Gain3/1 -> Sum5/2
  Sum/1 -> Uncertain State Space/1
  Demux/2 -> Sum4/1, Gain1/1
  Uncertain State Space1/1 -> Sum/1
  Sum2/1 -> Gain/1
  Sum1/1 -> Mux/1
  Sum5/1 -> Gain2/1

== system SDTlibV1/6 dof mechanisms/Revolute joint + configuration/18x18 v-u_rotation/Subsystem1 ==
  In1 : Inport
  Demux : Demux  Outputs=3
  Gain : Gain  Gain=2
  Gain1 : Gain  Gain=-2
  Gain2 : Gain  Gain=2
  Gain3 : Gain  Gain=2
  Gain4 : Gain  Gain=pass  Multiplication=Matrix(K*u) (u vector)
  Gain5 : Gain  Gain=pass'  Multiplication=Matrix(K*u) (u vector)
  Mux : Mux  Inputs=3
  Sum : Sum  Inputs=++|
  Sum1 : Sum  Inputs=|++
  Sum2 : Sum  Inputs=|+-
  Sum3 : Sum  Inputs=|++
  Sum4 : Sum  Inputs=++|
  Sum5 : Sum  Inputs=++|
  Uncertain State Space{,1..3} (4 alike) : RCTblocks/Uncertain State Space  Tag=USS  USystem=uss(sig4)  UValue=[]  X0=[]  uX0=[]
  Out1 : Outport  VectorParamsAs1DForOutWhenUnconnected=off
  wires:
  Gain5/1 -> Demux/1
  Sum5/1 -> Gain2/1
  Sum1/1 -> Mux/1
  Sum2/1 -> Gain/1
  Uncertain State Space1/1 -> Sum/1
  Demux/2 -> Gain1/1, Sum4/1
  Sum/1 -> Uncertain State Space/1
  Gain3/1 -> Sum5/2
  Uncertain State Space/1 -> Sum1/1, Sum5/1, Uncertain State Space1/1
  Gain1/1 -> Sum2/1
  Sum3/1 -> Uncertain State Space2/1
  Sum4/1 -> Mux/2
  Mux/1 -> Gain4/1
  Demux/3 -> Mux/3
  Demux/1 -> Sum1/2, Gain3/1
  Uncertain State Space2/1 -> Sum2/2, Sum4/2, Uncertain State Space3/1
  Gain/1 -> Sum/2
  In1/1 -> Gain5/1
  Gain2/1 -> Sum3/1
  Uncertain State Space3/1 -> Sum3/2
  Gain4/1 -> Out1/1

== system SDTlibV1/6 dof mechanisms/Revolute joint + configuration/18x18 v-u_rotation/Subsystem2 ==
  In1 : Inport
  Demux : Demux  Outputs=3
  Gain : Gain  Gain=2
  Gain1 : Gain  Gain=-2
  Gain2 : Gain  Gain=2
  Gain3 : Gain  Gain=2
  Gain4 : Gain  Gain=pass  Multiplication=Matrix(K*u) (u vector)
  Gain5 : Gain  Gain=pass'  Multiplication=Matrix(K*u) (u vector)
  Mux : Mux  Inputs=3
  Sum : Sum  Inputs=++|
  Sum1 : Sum  Inputs=|++
  Sum2 : Sum  Inputs=|+-
  Sum3 : Sum  Inputs=|++
  Sum4 : Sum  Inputs=++|
  Sum5 : Sum  Inputs=++|
  Uncertain State Space{,1..3} (4 alike) : RCTblocks/Uncertain State Space  Tag=USS  USystem=uss(sig4)  UValue=[]  X0=[]  uX0=[]
  Out1 : Outport  VectorParamsAs1DForOutWhenUnconnected=off
  wires:
  Sum5/1 -> Gain2/1
  Sum1/1 -> Mux/1
  Sum2/1 -> Gain/1
  Uncertain State Space1/1 -> Sum/1
  Demux/2 -> Gain1/1, Sum4/1
  Sum/1 -> Uncertain State Space/1
  Gain3/1 -> Sum5/2
  Uncertain State Space/1 -> Sum1/1, Sum5/1, Uncertain State Space1/1
  Gain1/1 -> Sum2/1
  Sum3/1 -> Uncertain State Space2/1
  Sum4/1 -> Mux/2
  Mux/1 -> Gain4/1
  Demux/3 -> Mux/3
  Demux/1 -> Sum1/2, Gain3/1
  Uncertain State Space2/1 -> Sum2/2, Sum4/2, Uncertain State Space3/1
  Gain/1 -> Sum/2
  In1/1 -> Gain5/1
  Gain2/1 -> Sum3/1
  Uncertain State Space3/1 -> Sum3/2
  Gain4/1 -> Out1/1
  Gain5/1 -> Demux/1

== system SDTlibV1/6 dof mechanisms/Revolute joint + configuration/18x18 v-u_rotation/Subsystem3 ==
  In1 : Inport
  Demux : Demux  Outputs=3
  Gain : Gain  Gain=2
  Gain1 : Gain  Gain=-2
  Gain2 : Gain  Gain=2
  Gain3 : Gain  Gain=2
  Gain4 : Gain  Gain=pass  Multiplication=Matrix(K*u) (u vector)
  Gain5 : Gain  Gain=pass'  Multiplication=Matrix(K*u) (u vector)
  Mux : Mux  Inputs=3
  Sum : Sum  Inputs=++|
  Sum1 : Sum  Inputs=|++
  Sum2 : Sum  Inputs=|+-
  Sum3 : Sum  Inputs=|++
  Sum4 : Sum  Inputs=++|
  Sum5 : Sum  Inputs=++|
  Uncertain State Space{,1..3} (4 alike) : RCTblocks/Uncertain State Space  Tag=USS  USystem=uss(sig4)  UValue=[]  X0=[]  uX0=[]
  Out1 : Outport  VectorParamsAs1DForOutWhenUnconnected=off
  wires:
  Gain4/1 -> Out1/1
  Uncertain State Space3/1 -> Sum3/2
  Gain2/1 -> Sum3/1
  In1/1 -> Gain5/1
  Gain/1 -> Sum/2
  Uncertain State Space2/1 -> Uncertain State Space3/1, Sum4/2, Sum2/2
  Demux/1 -> Gain3/1, Sum1/2
  Demux/3 -> Mux/3
  Mux/1 -> Gain4/1
  Sum4/1 -> Mux/2
  Sum3/1 -> Uncertain State Space2/1
  Gain1/1 -> Sum2/1
  Uncertain State Space/1 -> Uncertain State Space1/1, Sum5/1, Sum1/1
  Gain3/1 -> Sum5/2
  Sum/1 -> Uncertain State Space/1
  Demux/2 -> Sum4/1, Gain1/1
  Uncertain State Space1/1 -> Sum/1
  Sum2/1 -> Gain/1
  Sum1/1 -> Mux/1
  Sum5/1 -> Gain2/1
  Gain5/1 -> Demux/1

== system SDTlibV1/6 dof mechanisms/Revolute joint + configuration/18x18 v-u_rotation/Subsystem4 ==
  In1 : Inport
  Demux : Demux  Outputs=3
  Gain : Gain  Gain=2
  Gain1 : Gain  Gain=-2
  Gain2 : Gain  Gain=2
  Gain3 : Gain  Gain=2
  Gain4 : Gain  Gain=pass  Multiplication=Matrix(K*u) (u vector)
  Gain5 : Gain  Gain=pass'  Multiplication=Matrix(K*u) (u vector)
  Mux : Mux  Inputs=3
  Sum : Sum  Inputs=++|
  Sum1 : Sum  Inputs=|++
  Sum2 : Sum  Inputs=|+-
  Sum3 : Sum  Inputs=|++
  Sum4 : Sum  Inputs=++|
  Sum5 : Sum  Inputs=++|
  Uncertain State Space{,1..3} (4 alike) : RCTblocks/Uncertain State Space  Tag=USS  USystem=uss(sig4)  UValue=[]  X0=[]  uX0=[]
  Out1 : Outport  VectorParamsAs1DForOutWhenUnconnected=off
  wires:
  Gain5/1 -> Demux/1
  Gain4/1 -> Out1/1
  Uncertain State Space3/1 -> Sum3/2
  Gain2/1 -> Sum3/1
  In1/1 -> Gain5/1
  Gain/1 -> Sum/2
  Uncertain State Space2/1 -> Uncertain State Space3/1, Sum4/2, Sum2/2
  Demux/1 -> Gain3/1, Sum1/2
  Demux/3 -> Mux/3
  Mux/1 -> Gain4/1
  Sum4/1 -> Mux/2
  Sum3/1 -> Uncertain State Space2/1
  Gain1/1 -> Sum2/1
  Uncertain State Space/1 -> Uncertain State Space1/1, Sum5/1, Sum1/1
  Gain3/1 -> Sum5/2
  Sum/1 -> Uncertain State Space/1
  Demux/2 -> Sum4/1, Gain1/1
  Uncertain State Space1/1 -> Sum/1
  Sum2/1 -> Gain/1
  Sum1/1 -> Mux/1
  Sum5/1 -> Gain2/1
